simulink model "ZeroCrossing.v1"  (R2020a)
settings: Solver=VariableStepAuto  StartTime=0.0  StopTime=5  MaxStep=0.00001  RelTol=1e-3
settings Model: Creator=arne-  LastModifiedBy=arne-

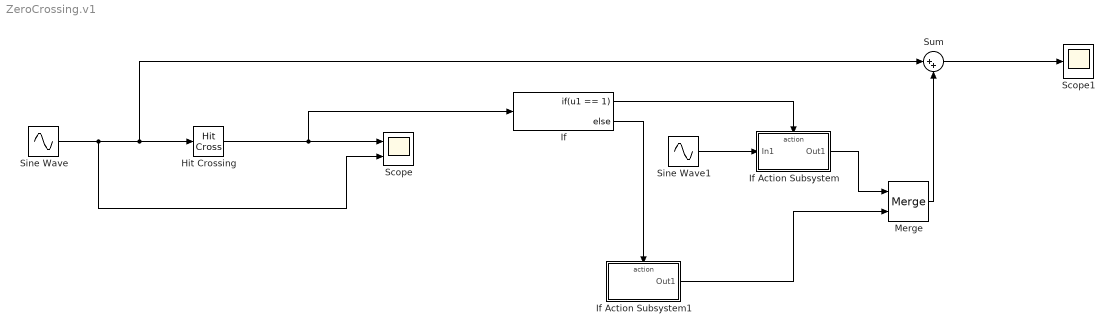
== system ZeroCrossing.v1 ==
  Hit Crossing : HitCross
  If : If  IfExpression=u1 == 1
  If Action Subsystem : Subsystem  TreatAsAtomicUnit=on
  If Action Subsystem1 : Subsystem  TreatAsAtomicUnit=on
  Merge : Merge
  Scope : Scope  NumInputPorts=2
  Scope1 : Scope
  Sine Wave : Sin  Amplitude=12.7  Frequency=314.16  SampleTime=0
  Sine Wave1 : Sin  Amplitude=2.5  Frequency=753982.236  SampleTime=0
  Sum : Sum  Inputs=|++
  wires:
  Hit Crossing/1 -> If/1, Scope/1
  Sine Wave/1 -> Scope/2, Sum/1, Hit Crossing/1
  If/1 -> If Action Subsystem/Action
  If/2 -> If Action Subsystem1/Action
  Sine Wave1/1 -> If Action Subsystem/1(In1)
  Sum/1 -> Scope1/1
  Merge/1 -> Sum/2
  If Action Subsystem/1(Out1) -> Merge/1
  If Action Subsystem1/1(Out1) -> Merge/2

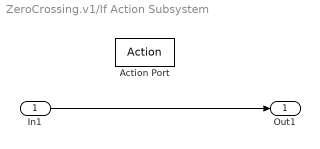
== system ZeroCrossing.v1/If Action Subsystem ==
  In1 : Inport
  Action Port : ActionPort  ActionPortLabel=if(u1 == 1)
  Out1 : Outport
  wires:
  In1/1 -> Out1/1

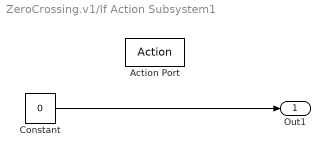
== system ZeroCrossing.v1/If Action Subsystem1 ==
  Action Port : ActionPort  ActionPortLabel=else
  Constant : Constant  Value=0
  Out1 : Outport
  wires:
  Constant/1 -> Out1/1
